simulink model "uwb_2_nature256"  (R2025a)
settings: Solver=VariableStepAuto  StartTime=0.0  StopTime=5e-8  RelTol=1e-3
undefined symbols (not defined in the file or in its folder): dspblkCoreblockFVToolHelper, gcbh
libraries: commdigbbndpm3 x2, commrfcorlib x1, simulink_extras x1, dspfiltersrcs x1, dspfdesign x1, simulink x1, dspsigops x1
settings Model: Creator=IWMAI  LastModifiedBy=IWMAI

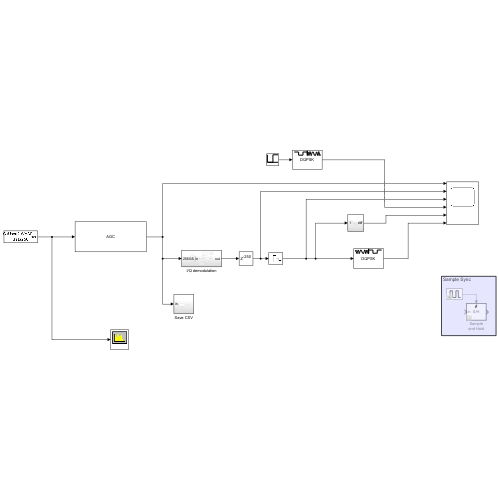
[thumbnail: Simulink's stored preview of the top-level diagram]
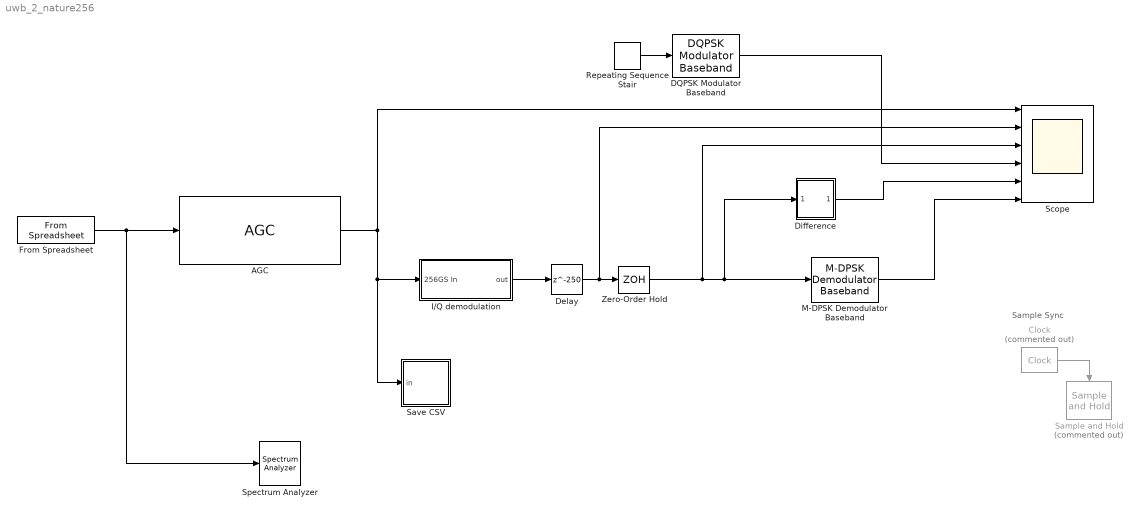
== system uwb_2_nature256 ==
  note: Sample Sync
  AGC : commrfcorlib/AGC  LegacyMode=off  DetectorMethod=Rectifier  LoopMethod=Linear  UpdatePeriod=100  StepSize=0.1  AdaptationStepSize=0.01  DesiredOutputPower=1  AveragingLength=1024  MaximumGain=30  MaxPowerGain=60  GainOutputPort=off  InputPowerOutputPort=off  SimulateUsing=Interpreted execution
  Clock : simulink_extras/Flip Flops/Clock  Commented=on  period=512.95 / 256e9
  DQPSK Modulator Baseband : commdigbbndpm3/DQPSK Modulator Baseband  InType=Integer  Enc=Gray  Ph=0  outDtype=double
  Delay : Delay  DelayLength=250
  Difference : Subsystem
  From Spreadsheet : FromSpreadsheet  FileName=C:\Users\IWMAI\University of Toronto\Yu Huang - Summer-2025-sharted\Yongkang\v3_250617\csv\data256.csv  SheetName=data256  OutDataTypeStr=double  SampleTime=1/256e9
  I/Q demodulation : Subsystem
  M-DPSK Demodulator Baseband : commdigbbndpm3/M-DPSK Demodulator Baseband  M=4  OutType=Integer  Dec=Gray  Ph=0  outDtype1=Inherit via internal rule  outDtype2=Inherit via internal rule
  Repeating Sequence Stair : simulink/Sources/Repeating Sequence Stair  OutValues=[0 2].'  tsamp=1/500003519.873597  OutMin=[]  OutMax=[]  OutDataTypeStr=double  OutputDataTypeScalingMode=double  OutDataType=fixdt(0,8)  ConRadixGroup=Best Precision: Vector-wise  OutScaling=2^-12
  Sample and Hold : dspsigops/Sample and Hold  Commented=on  trig=Rising edge  initCond=0  latchinput=off
  Save CSV : Subsystem
  Scope : Scope  NumInputPorts=6
      settings: ActiveDisplayYMinimum=-4.6231372013846705  ActiveDisplayYMaximum=4.7306324654418139
  Spectrum Analyzer : SpectrumAnalyzer  WindowPosition=[1050.000000,244.000000,800.000000,500.000000,]  Visible=on  ScopeFrameLocation=window  WindowInvariantSamplesPerUpdate=on  YLimits=[-60.8823 2.6232]
      settings: OpenAtSimulationStart=off
  Zero-Order Hold : ZeroOrderHold  SampleTime=1/500003519.873597
  wires:
  From Spreadsheet/1 -> Spectrum Analyzer/1, AGC/1
  I/Q demodulation/1(out) -> Delay/1
  Zero-Order Hold/1 -> Scope/3, M-DPSK Demodulator Baseband/1, Difference/1(In1)
  Clock/1 -> Sample and Hold/Trigger
  Repeating Sequence Stair/1 -> DQPSK Modulator Baseband/1
  Difference/1(diff) -> Scope/5
  AGC/1 -> Scope/1, Save CSV/1(in), I/Q demodulation/1(256GS In)
  M-DPSK Demodulator Baseband/1 -> Scope/6
  DQPSK Modulator Baseband/1 -> Scope/4
  Delay/1 -> Scope/2, Zero-Order Hold/1

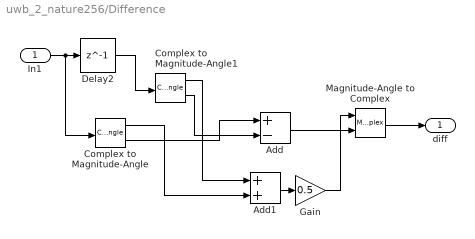
== system uwb_2_nature256/Difference ==
  In1 : Inport
  Add : Sum  Inputs=+-
  Add1 : Sum
  Complex to Magnitude-Angle : ComplexToMagnitudeAngle
  Complex to Magnitude-Angle1 : ComplexToMagnitudeAngle
  Delay2 : Delay  DelayLength=1
  Gain : Gain  Gain=0.5
  Magnitude-Angle to Complex : MagnitudeAngleToComplex
  diff : Outport
  wires:
  Gain/1 -> Magnitude-Angle to Complex/1
  Complex to Magnitude-Angle1/2 -> Add/2
  Add1/1 -> Gain/1
  Add/1 -> Magnitude-Angle to Complex/2
  Complex to Magnitude-Angle/2 -> Add/1
  Magnitude-Angle to Complex/1 -> diff/1
  Complex to Magnitude-Angle/1 -> Add1/2
  Complex to Magnitude-Angle1/1 -> Add1/1
  Delay2/1 -> Complex to Magnitude-Angle1/1
  In1/1 -> Delay2/1, Complex to Magnitude-Angle/1

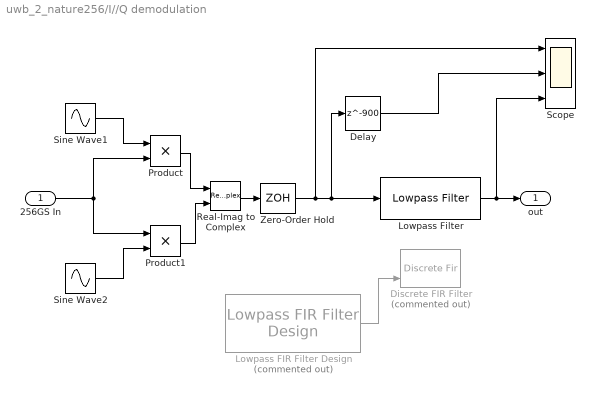
== system uwb_2_nature256/I//Q demodulation ==
  256GS In : Inport
  Delay : Delay  DelayLength=900
  Discrete FIR Filter : DiscreteFir  Commented=on  LoadFcn=dspblkCoreblockFVToolHelper(gcbh,'load');  CoefSource=Input port
      settings: CopyFcn=dspblkCoreblockFVToolHelper(gcbh,'copy');  DeleteFcn=dspblkCoreblockFVToolHelper(gcbh,'close');  ModelCloseFcn=dspblkCoreblockFVToolHelper(gcbh,'close');  PreSaveFcn=dspblkCoreblockFVToolHelper(gcbh,'presave');  PostSaveFcn=dspblkCoreblockFVToolHelper(gcbh,'postsave');  CloseFcn=dspblkCoreblockFVToolHelper(gcbh,'close');  InputPortMap=u0,u1
  Lowpass FIR Filter Design : dspfiltersrcs/Lowpass FIR Filter Design  Commented=on  SmoothParameters=off  SmoothingFactor=0.6  FilterOrderPort=off  FilterOrder=100  MaxOrder=100  CutoffFrequencyPort=off  CutoffFrequency=1/256e9  Window=Hann  SidelobeAttenuationPort=off  SidelobeAttenuation=60  KaiserWindowParameterPort=off  KaiserWindowParameter=.5  OutputDataType=double  SampleTime=1/256e9  SimulateUsing=Interpreted execution
      settings: LibrarySourceBlock=dspfdesign/Lowpass FIR Filter Design
  Lowpass Filter : dspfdesign/Lowpass Filter  FilterType=FIR  DesignForMinimumOrder=on  FilterOrder=50  PassbandFrequency=1/64  StopbandFrequency=1/32  PassbandRipple=0.1  StopbandAttenuation=80  SampleRateMode=Use normalized frequency (0 to 1)  SampleRate=44100  SimulateUsing=Interpreted execution  roundingMode=Floor  coeffsDataTypeStr=fixdt(1,16)
  Product : Product
  Product1 : Product
  Real-Imag to Complex : RealImagToComplex
  Scope : Scope  NumInputPorts=3
      settings: ActiveDisplayYMinimum=-3.8072894106917321  ActiveDisplayYMaximum=4.4801769671043541  DataLoggingVariableName=ScopeData2
  Sine Wave1 : Sin  Frequency=2 * pi * 4e9  Phase=pi/2  SampleTime=0
  Sine Wave2 : Sin  Frequency=2 * pi * 4e9  SampleTime=0
  Zero-Order Hold : ZeroOrderHold  SampleTime=1/256e9
  out : Outport
  wires:
  256GS In/1 -> Product/2, Product1/1
  Sine Wave2/1 -> Product1/2
  Sine Wave1/1 -> Product/1
  Product/1 -> Real-Imag to Complex/1
  Product1/1 -> Real-Imag to Complex/2
  Lowpass FIR Filter Design/1 -> Discrete FIR Filter/2
  Lowpass Filter/1 -> Scope/3, out/1
  Real-Imag to Complex/1 -> Zero-Order Hold/1
  Zero-Order Hold/1 -> Scope/1, Delay/1, Lowpass Filter/1
  Delay/1 -> Scope/2

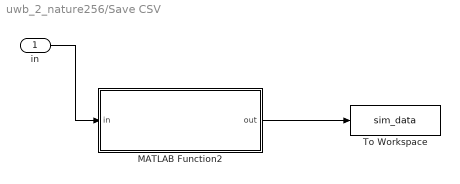
== system uwb_2_nature256/Save CSV ==
  in : Inport
  MATLAB Function2 : MATLAB Function  TreatAsAtomicUnit=on
  To Workspace : ToWorkspace  VariableName=sim_data  SaveFormat=Timeseries  SampleTime=-1
  wires:
  MATLAB Function2/1(out) -> To Workspace/1
  in/1 -> MATLAB Function2/1(in)

== matlab function uwb_2_nature256/Save CSV/MATLAB Function2 ==
  data: in input; out output
function out = save_csv(in)
%#codegen
% This function processes one sample at a time.
% To store data across simulation steps, you need to use persistent variables.

persistent data_buffer;
persistent index_counter;

if isempty(data_buffer)
    % Initialize buffer and counter when simulation starts or resets
    data_buffer = zeros(0, 2); % Column 1 for index, Column 2 for data
    index_counter = 0;
end

% Increment index and store current sample
index_counter = index_counter + 1;
data_buffer = [data_buffer; index_counter, in];

% Output the current sample (or anything else you need downstream)
out = in;

% You can add logic here to write to CSV periodically,
% but it's generally better to do it after simulation.
% For this method, we'll let 'To Workspace' handle saving.

% At the end of simulation, the persistent variables will be cleared unless
% you explicitly save them or access them from the base workspace.
% For 'To Workspace' method, it's about the *output* of this block.
end
